simulink model "MainDriveCoolingEx"  (Simulink 7.6)
settings: Solver=ode45  StartTime=0.0  StopTime=10.0  RelTol=1e-3
undefined symbols (not defined in the file or in its folder): A, epsilon, R
settings Model: Creator=conid  LastModifiedBy=conid

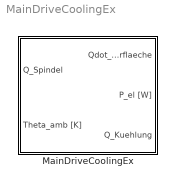
== system MainDriveCoolingEx ==
  MainDriveCoolingEx : Subsystem

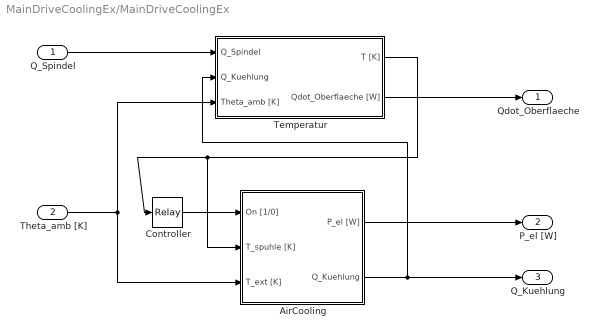
== system MainDriveCoolingEx/MainDriveCoolingEx ==
  Q_Spindel : Inport
  Theta_amb [K] : Inport  Port=2
  AirCooling : Subsystem
  Controller : Relay
  Temperatur : Subsystem
  Qdot_Oberflaeche : Outport
  P_el [W] : Outport  Port=2
  Q_Kuehlung : Outport  Port=3
  wires:
  Controller/1 -> AirCooling/1(On [1/0])
  Temperatur/1(T [K]) -> Controller/1, AirCooling/2(T_spuhle [K])
  Theta_amb [K]/1 -> Temperatur/3(Theta_amb [K]), AirCooling/3(T_ext [K])
  Q_Spindel/1 -> Temperatur/1(Q_Spindel)
  AirCooling/2(Q_Kuehlung) -> Q_Kuehlung/1, Temperatur/2(Q_Kuehlung)
  AirCooling/1(P_el [W]) -> P_el [W]/1
  Temperatur/2(Qdot_Oberflaeche [W]) -> Qdot_Oberflaeche/1

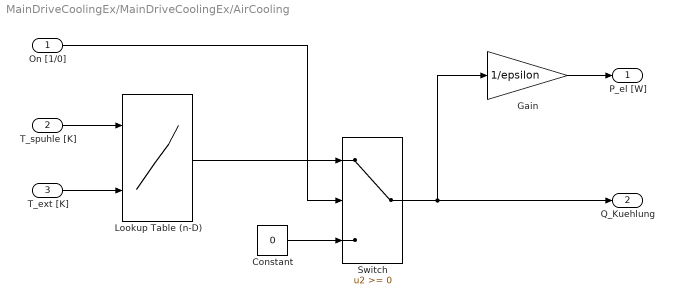
== system MainDriveCoolingEx/MainDriveCoolingEx/AirCooling ==
  On [1/0] : Inport
  T_spuhle [K] : Inport  Port=2
  T_ext [K] : Inport  Port=3
  Constant : Constant  Value=0
  Gain : Gain  Gain=1/epsilon
  Lookup Table (n-D) : Lookup_n-D  InputSameDT=on
  Switch : Switch
  P_el [W] : Outport
  Q_Kuehlung : Outport  Port=2
  wires:
  Gain/1 -> P_el [W]/1
  Switch/1 -> Q_Kuehlung/1, Gain/1
  Lookup Table (n-D)/1 -> Switch/1
  Constant/1 -> Switch/3
  On [1/0]/1 -> Switch/2
  T_spuhle [K]/1 -> Lookup Table (n-D)/1
  T_ext [K]/1 -> Lookup Table (n-D)/2

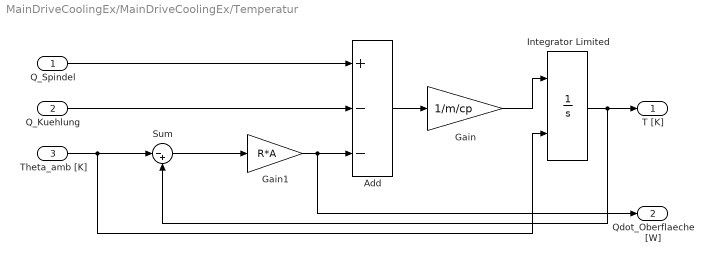
== system MainDriveCoolingEx/MainDriveCoolingEx/Temperatur ==
  Q_Spindel : Inport
  Q_Kuehlung : Inport  Port=2
  Theta_amb [K] : Inport  Port=3
  Add : Sum  Inputs=+--
  Gain : Gain  Gain=1/m/cp
  Gain1 : Gain  Gain=R*A
  Integrator Limited : Integrator  InitialConditionSource=external  LimitOutput=on  ZeroCross=off
  Sum : Sum  Inputs=|-+
  T [K] : Outport
  Qdot_Oberflaeche [W] : Outport  Port=2
  wires:
  Add/1 -> Gain/1
  Gain/1 -> Integrator Limited/1
  Integrator Limited/1 -> T [K]/1, Sum/2
  Sum/1 -> Gain1/1
  Gain1/1 -> Add/3, Qdot_Oberflaeche [W]/1
  Q_Spindel/1 -> Add/1
  Theta_amb [K]/1 -> Sum/1, Integrator Limited/2
  Q_Kuehlung/1 -> Add/2
